simulink model "SPWM"  (R2024b)
settings: Solver=VariableStepAuto  StartTime=0.0  StopTime=0.08  RelTol=1e-3
model workspace (MAT data in the model file):
  f = Simulink.Parameter
  f.Complexity = 'real'
  f.Dimensions = [0 0]
  f.DataType = 'auto'
libraries: spsOnDelayLib x6, spsThreePhaseSeriesRLCBranchLib x3, spsVoltageMeasurementLib x2, spsDCVoltageSourceLib x1, spsUniversalBridgeLib x1, sps_lib x1, spsTriangleGeneratorLib x1, spsCurrentMeasurementLib x1
settings Model: Creator=42971  LastModifiedBy=42971
settings DataIOCC: ReturnWorkspaceOutputs=off

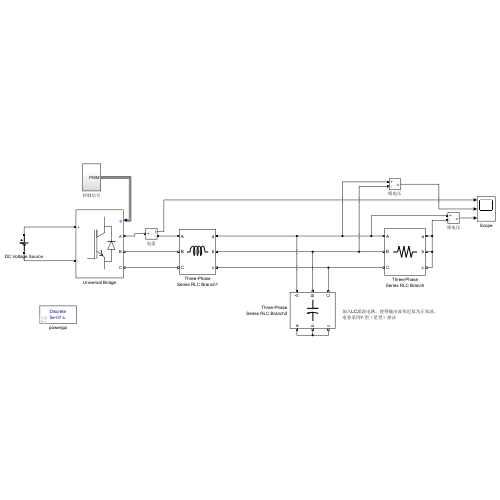
[thumbnail: Simulink's stored preview of the top-level diagram]
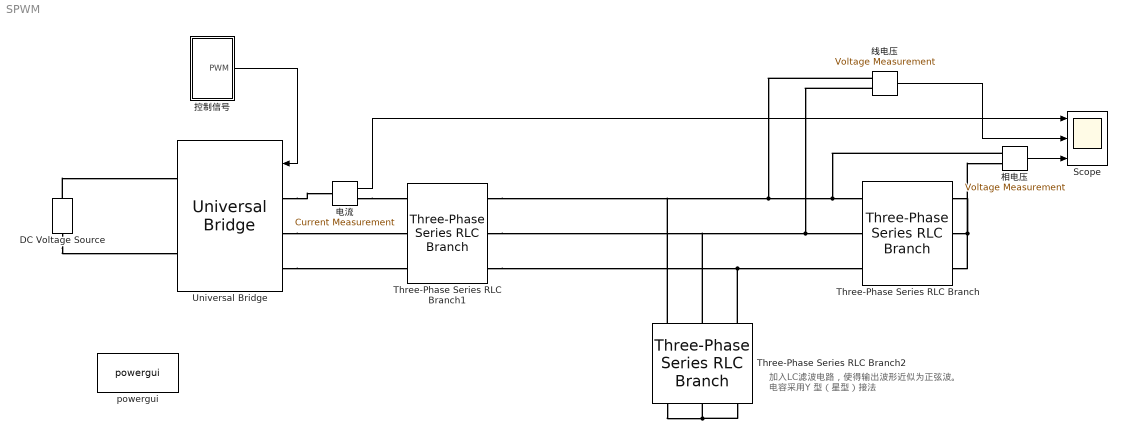
== system SPWM ==
  note: 加入LC滤波电路，使得输出波形近似为正弦波。
      | 电容采用Y 型（星型）接法
  DC Voltage Source : spsDCVoltageSourceLib/DC Voltage Source  Amplitude=200  Measurements=None
  Scope : Scope  NumInputPorts=3
  Three-Phase Series RLC Branch : spsThreePhaseSeriesRLCBranchLib/Three-Phase Series RLC Branch  LConnTagsString=A|B|C  RConnTagsString=A|B|C  BranchType=R  Resistance=20  Inductance=0.01  Capacitance=0  Measurements=None
  Three-Phase Series RLC Branch1 : spsThreePhaseSeriesRLCBranchLib/Three-Phase Series RLC Branch  LConnTagsString=A|B|C  RConnTagsString=A|B|C  BranchType=L  Resistance=0.0000001  Inductance=4.501e-3  Capacitance=0  Measurements=None
  Three-Phase Series RLC Branch2 : spsThreePhaseSeriesRLCBranchLib/Three-Phase Series RLC Branch  LConnTagsString=A|B|C  RConnTagsString=A|B|C  BranchType=C  Resistance=20  Inductance=0.01  Capacitance=1.0026e-5  Measurements=None
  Universal Bridge : spsUniversalBridgeLib/Universal Bridge  Arms=3  SnubberResistance=1e5  SnubberCapacitance=inf  Device=IGBT / Diodes  Ron=1e-3  Lon=0  ForwardVoltages="[  0  0  ]"  ForwardVoltage=0  GTOparameters=[ 10e-6 , 20e-6 ]  IGBTparameters=[ 1e-6 , 2e-6 ]  Measurements=None  Measurements_2=None  converterType=Rectifier
  powergui : sps_lib/powergui  Priority=1  SimulationMode=Discrete  SampleTime=5e-7  frequency=60  Iterations=50  frequencyindice=0  Pbase=100e6  ErrMax=1e-4  UnitsV=kV  UnitsW=MW  buscounter=0  FunctionMessages=off  echomessages=off  EnableUseOfTLC=off  CurrentSourceSwitches=off  DisableSnubberDevices=off  DisableRonSwitches=off  DisableVfSwitches=off  DisplayEquations=off  AutomaticDiscreteSolvers=off  SolverType=Tustin/Backward Euler (TBE)  Interpol=off  ExternalGateDelay=off  methode=off  Ts=100  x0status=blocks  SPID=on  SwTol=0  HookPort=off  NonlinearTolerance=1e-4  nMaxIteration=100  ContinueOnMaxIteration=off  RestoreLinks=warning  ResistiveCurrentMeasurement=off  Frange=[0:2:500]  Ylog=off  Xlog=on  ShowGrid=off  save=off  variable=ZData  structure=0  ZoomFFT=off  StartTime=0.0  cycles=1  DisplayStyle=1  fundamental=60  FreqAxis=off  MaxFrequency=1000  frequencyindicesteady=1  RmsSteady=1  display=off
  控制信号 : Subsystem
  电流 : spsCurrentMeasurementLib/Current Measurement  PhasorSimulation=off  OutputType=Complex  PSBequivalent=0
  相电压 : spsVoltageMeasurementLib/Voltage Measurement  PhasorSimulation=off  OutputType=Complex  PSBequivalent=0
  线电压 : spsVoltageMeasurementLib/Voltage Measurement  PhasorSimulation=off  OutputType=Complex  PSBequivalent=0
  wires:
  相电压/1 -> Scope/3
  线电压/1 -> Scope/2
  控制信号/1(PWM) -> Universal Bridge/1
  电流/1 -> Scope/1
  connections:
  Universal Bridge/LConn1 -- 电流/LConn1
  线电压/LConn2 -- Three-Phase Series RLC Branch1/RConn2 -- Three-Phase Series RLC Branch2/LConn2 -- Three-Phase Series RLC Branch/LConn2
  Three-Phase Series RLC Branch/RConn2 -- Three-Phase Series RLC Branch/RConn3 -- Three-Phase Series RLC Branch/RConn1 -- 相电压/LConn2
  线电压/LConn1 -- Three-Phase Series RLC Branch1/RConn1 -- Three-Phase Series RLC Branch2/LConn1 -- 相电压/LConn1 -- Three-Phase Series RLC Branch/LConn1
  DC Voltage Source/RConn1 -- Universal Bridge/RConn1
  DC Voltage Source/LConn1 -- Universal Bridge/RConn2
  Universal Bridge/LConn2 -- Three-Phase Series RLC Branch1/LConn2
  Universal Bridge/LConn3 -- Three-Phase Series RLC Branch1/LConn3
  电流/RConn1 -- Three-Phase Series RLC Branch1/LConn1
  Three-Phase Series RLC Branch2/LConn3 -- Three-Phase Series RLC Branch/LConn3 -- Three-Phase Series RLC Branch1/RConn3
  Three-Phase Series RLC Branch2/RConn1 -- Three-Phase Series RLC Branch2/RConn3 -- Three-Phase Series RLC Branch2/RConn2

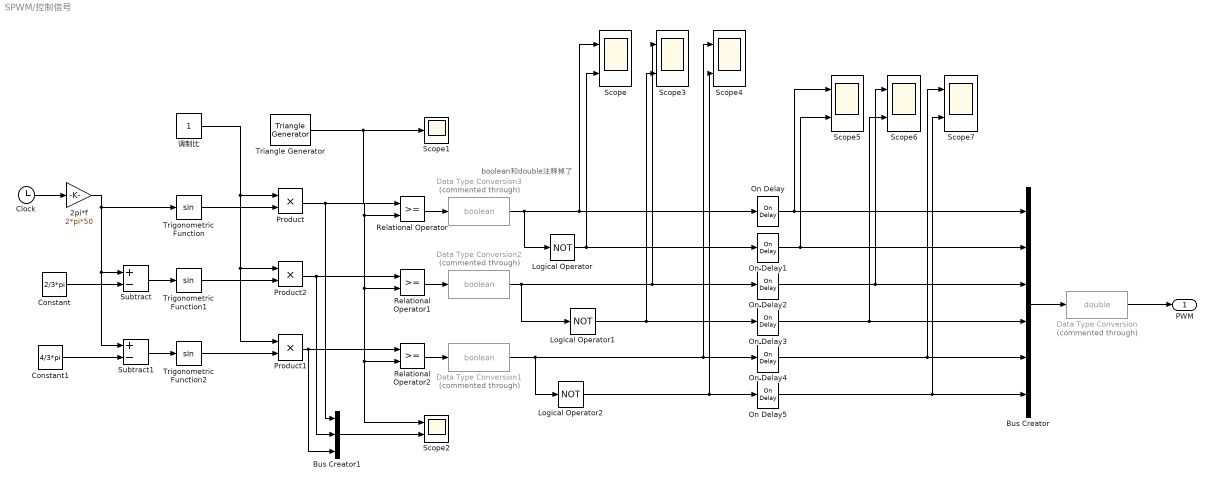
== system SPWM/控制信号 ==
  note: boolean和double注释掉了
  2pi*f : Gain  Gain=2*pi*50
  Bus Creator : BusCreator  Inputs=6
  Bus Creator1 : BusCreator  Inputs=3
  Clock : Clock
  Constant : Constant  Value=2/3*pi
  Constant1 : Constant  Value=4/3*pi
  Data Type Conversion : DataTypeConversion  Commented=through  OutDataTypeStr=double  SaturateOnIntegerOverflow=off  RndMeth=Floor
  Data Type Conversion1 : DataTypeConversion  Commented=through  OutDataTypeStr=boolean  SaturateOnIntegerOverflow=off  RndMeth=Floor
  Data Type Conversion2 : DataTypeConversion  Commented=through  OutDataTypeStr=boolean  SaturateOnIntegerOverflow=off  RndMeth=Floor
  Data Type Conversion3 : DataTypeConversion  Commented=through  OutDataTypeStr=boolean  SaturateOnIntegerOverflow=off  RndMeth=Floor
  Logical Operator : Logic  Operator=NOT  AllPortsSameDT=off  OutDataTypeStr=boolean
  Logical Operator1 : Logic  Operator=NOT  AllPortsSameDT=off  OutDataTypeStr=boolean
  Logical Operator2 : Logic  Operator=NOT  AllPortsSameDT=off  OutDataTypeStr=boolean
  On Delay{,1..5} (6 alike) : spsOnDelayLib/On Delay  DelayType=On delay  delay=2e-6  ic=0  Ts=0
  Product : Product
  Product1 : Product
  Product2 : Product
  Relational Operator : RelationalOperator  OutDataTypeStr=boolean  RndMeth=Simplest  InputSameDT=off
  Relational Operator1 : RelationalOperator  OutDataTypeStr=boolean  RndMeth=Simplest  InputSameDT=off
  Relational Operator2 : RelationalOperator  OutDataTypeStr=boolean  RndMeth=Simplest  InputSameDT=off
  Scope{,2..7} (7 alike) : Scope  NumInputPorts=2
  Scope1 : Scope
  Subtract : Sum  Inputs=+-
  Subtract1 : Sum  Inputs=+-
  Triangle Generator : spsTriangleGeneratorLib/Triangle Generator  Freq=10000  Phase=0  Ts=1e-6
  Trigonometric Function : Trigonometry
  Trigonometric Function1 : Trigonometry
  Trigonometric Function2 : Trigonometry
  调制比 : Constant
  PWM : Outport
  wires:
  Trigonometric Function/1 -> Product/2
  Data Type Conversion1/1 -> On Delay4/1, Scope4/1, Logical Operator2/1
  Trigonometric Function2/1 -> Product1/2
  Data Type Conversion3/1 -> On Delay/1, Scope/1, Logical Operator/1
  Data Type Conversion2/1 -> Logical Operator1/1, On Delay2/1, Scope3/1
  Relational Operator2/1 -> Data Type Conversion1/1
  Logical Operator1/1 -> On Delay3/1, Scope3/2
  Subtract/1 -> Trigonometric Function1/1
  Product/1 -> Bus Creator1/1, Relational Operator/1
  Relational Operator/1 -> Data Type Conversion3/1
  2pi*f/1 -> Subtract/1, Subtract1/1, Trigonometric Function/1
  Product2/1 -> Bus Creator1/2, Relational Operator1/1
  Bus Creator1/1 -> Scope2/2
  Subtract1/1 -> Trigonometric Function2/1
  Triangle Generator/1 -> Scope1/1, Scope2/1, Relational Operator2/2, Relational Operator1/2, Relational Operator/2
  调制比/1 -> Product1/1, Product2/1, Product/1
  Bus Creator/1 -> Data Type Conversion/1
  Trigonometric Function1/1 -> Product2/2
  Relational Operator1/1 -> Data Type Conversion2/1
  Clock/1 -> 2pi*f/1
  Constant/1 -> Subtract/2
  Product1/1 -> Bus Creator1/3, Relational Operator2/1
  Constant1/1 -> Subtract1/2
  Logical Operator/1 -> On Delay1/1, Scope/2
  Data Type Conversion/1 -> PWM/1
  Logical Operator2/1 -> On Delay5/1, Scope4/2
  On Delay/1 -> Scope5/1, Bus Creator/1
  On Delay1/1 -> Scope5/2, Bus Creator/2
  On Delay2/1 -> Scope6/1, Bus Creator/3
  On Delay3/1 -> Scope6/2, Bus Creator/4
  On Delay4/1 -> Scope7/1, Bus Creator/5
  On Delay5/1 -> Scope7/2, Bus Creator/6
